simulink model "eVTOL_HIL"  (R2024b)
settings: Solver=FixedStepAuto  StartTime=0.0  StopTime=inf  FixedStep=SAMPLE_TIME  RelTol=1e-3
values from neighbouring files (symbols this model uses):
  aDl =     [initdata.mat]
  aDr =     [initdata.mat]
  aDyn =     [initdata.mat]
  aLat =     [initdata.mat]
  aLon =     [initdata.mat]
  D = Prop.D    [EOM_dt_MC.m]    (also in EOM_get_alf_dt_de_prop_evtol.m = CD * QS)
  General = init_layoutdata    [EOM_dt_MC.m]    (also in build_optimized_CA.m; initdata.mat = ; initdata_HIL_eVTOL.m)
  mass = Con(3)    [EOM_get_alf_dt_de_prop_evtol.m]    (also in initdata.mat = 2255.54; initdata_HIL_eVTOL.m = 7)
  Motor = init_motor_evtol    [EOM_dt_MC.m]    (also in initdata.mat = []; initdata_HIL_eVTOL.m)
  Prop = init_propeller_evtol_new    [EOM_dt_MC.m]    (also in initdata_HIL_eVTOL.m)
  SAMPLE_TIME = 0.01    [initdata_HIL_eVTOL.m]
undefined symbols (not defined in the file or in its folder): aDa, aDe, asbhl20env, Environment, InitData, magnitude
libraries: simulink_extras x16, vrlib x8, matrix_library x6, sharedutil x6, aerolibwindfilters x4, sharedtransform x4, aerolibfltsims x3, instrumentseriallib x3, uavmavlinklib x3, aerolibasang x3, aerolibobsolete x2, aerolibanimutils x1
(part 2 of 4)

== system eVTOL_HIL/eVTOL Dynamic Model/Environment/Wind Models ==
  Xe_x : Inport
  Ve : Inport  Port=2
  Altitude : Inport  Port=3
  DCM : Inport  Port=4
  Constant1 : Constant  Value=[0,0,0]
  Constant2 : Constant  Value=[0,0,0]
  Dot Product1 : DotProduct  OutDataTypeStr=Inherit: Inherit via internal rule
  Dot Product2 : DotProduct  OutDataTypeStr=Inherit: Inherit via internal rule
  Dryden Wind Turbulence Model (Continuous (+q -r)) : Subsystem  AncestorBlock=|  mask(Wind Turbulence Model){units=Metric (MKS), spec=MIL-F-8785C, model=Continuous Dryden (+q -r), W20=8, Wdeg=0, TurbProb=10^-4, L_high=533.4, Wingspan=7, ts=0.01, Seed=[23341 23342 23343 23344], T_on=on}
      | CustomLib_2019b/Dryden Wind Turbulence Model 
      | (Continuous (+q -r))
      mask prompts: units "aeroblks:aeroblkwind:blockWindTurbulenceModelParamUnits"; spec "aeroblks:aeroblkwind:blockWindTurbulenceModelParamSpecification"; model "aeroblks:aeroblkwind:blockWindTurbulenceModelParamModeltype"; W20 "Wind speed at 6 m defines the low-altitude intensity (m/s):"; Wdeg "Wind direction at 6 m (degrees clockwise from north):"; TurbProb "aeroblks:aeroblkwind:blockWindTurbulenceModelParamProbabilityofexceedanceofhighaltitudeintensity"; L_high "Scale length at medium/high altitudes (m):"; Wingspan "Wingspan (m):"; ts "Band limited noise sample time (sec):"; Seed "aeroblks:aeroblkwind:blockWindTurbulenceModelParamNoiseseedsugvgwgpg"; T_on "aeroblks:aeroblkwind:blockWindTurbulenceModelParamTurbulenceon"
      mask help: aeroblks:aeroblkwind:blockWindTurbulenceModelDesc
      mask init:
      | index = strfind(model,' ');
      | disp1 = model(1:index(1)-1);
      | disp2 = model(index(1)+1:index(end-1)-1);
      | disp3 = model(index(end-1)+1:end);
      | 
      | h_vec = [.5 1.75 3.75 7.5 15 25 35 45 55 65 75 80]*1000;% feet
      | sigma_vec(1,:) = [3.2 2.2 1.5 zeros(1,9)]; % ft/sec
      | sigma_vec(2,:) = [4.2 3.6 3.3 1.6 zeros(1,8)];
      | sigma_vec(3,:) = [6.6 6.9 7.4 6.7 4.6 2.7 0.4 zeros(1,5)];
      | sigma_vec(4,:) = [8.6 9.6 10.6 10.1 8.0 6.6 5.0 4.2 2.7 zeros(1,3)];
      | sigma_vec(5,:) = [11.8 13.0 16.0 15.1 11.6 9.7 8.1 8.2 7.9 4.9 3.2 2.1];
      | sigma_vec(6,:) = [15.6 17.6 23.0 23.6 22.1 20.0 16.0 15.1 12.1 7.9 6.2 5.1];
      | sigma_vec(7,:) = [18.7 21.5 28.4 30.2 30.7 31.0 25.2 23.1 17.5 10.7 8.4 7.2];
      | max_height_low = 1000;
      | if strcmp(spec,'MIL-F-8785C')
      |     min_height_high = 2000;
      | else
      | 	min_height_high = 1750;
      | end
      | [ports] = aeroicon('aeroblkwindturb2','icon');
      | 
      | dt=ts;
      settings: LibrarySourceBlock=|
      | CustomLib_2019b/Dryden Wind Turbulence Model
      | (Continuous (+q -r))
      mask Help: eval('asbhelp(''Dryden Wind Turbulence Model (Continuous)'')');
      mask TypeOptions units: aeroblks:aeroblkwind:blockWindTurbulenceModelParamComboMetricMKS | aeroblks:aeroblkwind:blockWindTurbulenceModelParamComboEnglishVelocityinfts | aeroblks:aeroblkwind:blockWindTurbulenceModelParamComboEnglishVelocityinkts
      mask TypeOptions spec: aeroblks:aeroblkwind:blockWindTurbulenceModelParamComboMILF8785C | aeroblks:aeroblkwind:blockWindTurbulenceModelParamComboMILHDBK1797 | aeroblks:aeroblkwind:blockWindTurbulenceModelParamComboMILHDBK1797B
      mask TypeOptions model: aeroblks:aeroblkwind:blockWindTurbulenceModelParamComboContinuousVonKarmanqr1 | aeroblks:aeroblkwind:blockWindTurbulenceModelParamComboContinuousVonKarmanqr2 | aeroblks:aeroblkwind:blockWindTurbulenceModelParamComboContinuousVonKarmanqr3 | aeroblks:aeroblkwind:blockWindTurbulenceModelParamComboContinuousDrydenqr1 | aeroblks:aeroblkwind:blockWindTurbulenceModelParamComboContinuousDrydenqr2 | aeroblks:aeroblkwind:blockWindTurbulenceModelParamComboContinuousDrydenqr3 | aeroblks:aeroblkwind:blockWindTurbulenceModelParamComboDiscreteDrydenqr1 | aeroblks:aeroblkwind:blockWindTurbulenceModelParamComboDiscreteDrydenqr2 | aeroblks:aeroblkwind:blockWindTurbulenceModelParamComboDiscreteDrydenqr3
      mask Callback model: aeroicon('aeroblkwindturb2');
      mask TypeOptions TurbProb: aeroblks:aeroblkwind:blockWindTurbulenceModelParamCombo2x101 | aeroblks:aeroblkwind:blockWindTurbulenceModelParamCombo101 | aeroblks:aeroblkwind:blockWindTurbulenceModelParamCombo102Light | aeroblks:aeroblkwind:blockWindTurbulenceModelParamCombo103Moderate | aeroblks:aeroblkwind:blockWindTurbulenceModelParamCombo104 | aeroblks:aeroblkwind:blockWindTurbulenceModelParamCombo105Severe | aeroblks:aeroblkwind:blockWindTurbulenceModelParamCombo106
      mask DialogControl units Prompt: Units:
      mask DialogControl spec Prompt: Specification:
      mask DialogControl model Prompt: Model type:
      mask DialogControl TurbProb Prompt: Probability of exceedance of high-altitude intensity:
      mask DialogControl Seed Prompt: Noise seeds [ug vg wg pg]:
      mask DialogControl T_on Prompt: Turbulence on
      mask Display:
      | port_label(ports(1).type,ports(1).port,ports(1).txt,'texmode','on');
      | port_label(ports(2).type,ports(2).port,ports(2).txt,'texmode','on');
      | port_label(ports(3).type,ports(3).port,ports(3).txt,'texmode','on');
      | port_label(ports(4).type,ports(4).port,ports(4).txt,'texmode','on');
      | port_label(ports(5).type,ports(5).port,ports(5).txt,'texmode','on');
  Gain4 : Gain  Gain=[1,1,1]
  Manual Switch1 : ManualSwitch  CurrentSetting=0
  Manual Switch2 : ManualSwitch  CurrentSetting=0
  Sqrt : Sqrt
  vt1 : Math  Operator=sqrt  SignedPower=on
  wind scp2 : Scope
  wind_mag scp : Scope
  windangular scp : Scope
  windspeed scp : Scope
  ug,vg,wg1 : Outport  VectorParamsAs1DForOutWhenUnconnected=off
  pg,qg,rg1 : Outport  Port=2  VectorParamsAs1DForOutWhenUnconnected=off
  wires:
  Manual Switch2/1 -> ug,vg,wg1/1  "WindVelocity"
  Dryden Wind Turbulence Model (Continuous (+q -r))/1(ug,vg,wg) -> Gain4/1, windspeed scp/1, Dot Product2/2, Dot Product2/1  "Vw"
  Dryden Wind Turbulence Model (Continuous (+q -r))/2(pg,qg,rg) -> Manual Switch1/1, windangular scp/1  "WindAngularRates"
  Constant1/1 -> Manual Switch1/2
  Altitude/1 -> [Altitude]
  vt1/1 -> [Airspeed]  "Airspeed"
  Constant2/1 -> Manual Switch2/2
  [Airspeed] -> Dryden Wind Turbulence Model (Continuous (+q -r))/2(Airspeed)  "Airspeed"
  DCM/1 -> [DCM]
  Ve/1 -> Dot Product1/2, Dot Product1/1
  Manual Switch1/1 -> pg,qg,rg1/1  "WindAngularRates"
  Gain4/1 -> Manual Switch2/1  "WindVelocity"
  [Altitude] -> Dryden Wind Turbulence Model (Continuous (+q -r))/1(Altitude)
  Dot Product2/1 -> Sqrt/1
  [DCM] -> Dryden Wind Turbulence Model (Continuous (+q -r))/3(DCM)
  Dot Product1/1 -> vt1/1
  Sqrt/1 -> wind_mag scp/1  "wind_mag"
  Xe_x/1 -> [x]
  [x] -> wind scp2/1

== system eVTOL_HIL/eVTOL Dynamic Model/airframe/Flight Conditions ==
  EnvData : Inport
  UAVData : Inport  Port=2
  Bus Selector : BusSelector  OutputSignals=Ve,Xe,Vb,pqr
  Bus Selector1 : BusSelector  OutputSignals=WindVelocity,WindAngularRate,T(K),a,Air_pressure,Air_density,g
  Constant : Constant  Value=0
  Demux1 : Demux  Outputs=2
  Derivative : Derivative
  Dynamic Pressure : aerolibasang/Dynamic Pressure
  Flat Earth to LLA : FlatEarth2LLA  R=6378137  LL0=[InitData.lat_deg, InitData.lon_deg]
  Gain : Gain  Gain=1/1.225
  "Incidence, Sideslip, & Airspeed" : aerolibasang/Incidence, Sideslip, & Airspeed
  MATLAB Function : MATLAB Function  TreatAsAtomicUnit=on
  Mach Number : aerolibasang/Mach Number
  Product : Product
  Sqrt : Sqrt
  Subsystem2 : Subsystem
  Sum : Sum  Inputs=|+-
  Sum1 : Sum  Inputs=|+-
  Vel in Inertial Axes : Subsystem
  lat_deg : Outport
  lon_deg : Outport  Port=2
  AMSL : Outport  Port=3
  gamma : Outport  Port=4
  chi : Outport  Port=5
  alphaDot : Outport  Port=6
  alpha : Outport  Port=7
  beta : Outport  Port=8
  TAS : Outport  Port=9
  pqr_air : Outport  Port=10
  Mach : Outport  Port=11
  DynamicPressure : Outport  Port=12
  EAS : Outport  Port=13
  T(K) : Outport  Port=14
  Air_pressure : Outport  Port=15
  g : Outport  Port=16
  Vb_air : Outport  Port=17
  Ve_Inertial : Outport  Port=18
  wires:
  Bus Selector/3 -> Sum/1  "<Vb>"
  Subsystem2/2(chi) -> chi/1  "chi"
  "Incidence, Sideslip, & Airspeed"/1 -> alpha/1, Derivative/1  "alpha"
  Subsystem2/1(gamma) -> gamma/1  "gamma"
  Demux1/1 -> lat_deg/1  "lat_deg"
  Bus Selector/2 -> Flat Earth to LLA/1  "<Xe>"
  Constant/1 -> Flat Earth to LLA/2
  Sum1/1 -> pqr_air/1  "pqr_air"
  Gain/1 -> Sqrt/1
  Flat Earth to LLA/2 -> AMSL/1  "AMSL"
  Product/1 -> EAS/1  "EAS"
  Bus Selector1/7 -> g/1  "<g>"
  Mach Number/1 -> Mach/1  "Mach"
  Bus Selector/4 -> Sum1/1  "<pqr>"
  UAVData/1 -> Bus Selector/1
  "Incidence, Sideslip, & Airspeed"/3 -> Product/1, TAS/1  "TAS"
  Bus Selector1/5 -> Air_pressure/1  "<Air_pressure>"
  Bus Selector1/6 -> Gain/1, Dynamic Pressure/2  "<Air_density>"
  Vel in Inertial Axes/1(Ve_Inertial) -> Ve_Inertial/1  "Ve_Inertial"
  Sum/1 -> "Incidence, Sideslip, & Airspeed"/1, Mach Number/1, Dynamic Pressure/1, MATLAB Function/1(u)  "Vb_air"
  Bus Selector1/3 -> T(K)/1  "<T(K)>"
  Derivative/1 -> alphaDot/1  "alphaDot"
  Bus Selector1/1 -> Sum/2  "<WindVelocity>"
  "Incidence, Sideslip, & Airspeed"/2 -> beta/1  "beta"
  Bus Selector/1 -> Vel in Inertial Axes/1(Ve), Subsystem2/1(Ve)  "<Ve>"
  Dynamic Pressure/1 -> DynamicPressure/1  "DynamicPressure"
  EnvData/1 -> Bus Selector1/1
  Bus Selector1/4 -> Mach Number/2  "<a>"
  Bus Selector1/2 -> Sum1/2  "<WindAngularRate>"
  Demux1/2 -> lon_deg/1  "lon_deg"
  Flat Earth to LLA/1 -> Demux1/1
  Sqrt/1 -> Product/2
  MATLAB Function/1(y) -> Vb_air/1

== system eVTOL_HIL/eVTOL Dynamic Model/airframe/force moment ==
  note: force and moment in body fixed axis coordination
  PlantData : Inport
  Act_surface : Inport  Port=2
  prop : Inport  Port=3
  EnvmData : Inport  Port=4
  Add : Sum  Inputs=++++
  Add1 : Sum  Inputs=++++
  Disturbance : Constant  Value=[0,10,0]
  Disturbance1 : Constant  Value=[0,0,0]
  F_Gear_in_b scp : Scope  Commented=on
  Gear&FM in body axis : Subsystem  Commented=on
  M_Gear scp : Scope  Commented=on
  Manual Switch : ManualSwitch  CurrentSetting=0
  Motor moment scp : Scope
  Scope{,1..4,6} (6 alike) : Scope
  Thrust&M in body axis : Subsystem
  aero F&M in body axis : Subsystem
  gravity in body axis : Subsystem
  Fb (X Y Z) : Outport  VectorParamsAs1DForOutWhenUnconnected=off
  M (L M N) : Outport  Port=2  VectorParamsAs1DForOutWhenUnconnected=off
  wires:
  Thrust&M in body axis/1(f_T) -> Add/1, Scope4/1
  gravity in body axis/1(Fb) -> Add/3, Scope3/1
  Thrust&M in body axis/2(m_T) -> Add1/1, Motor moment scp/1
  aero F&M in body axis/2(M (L M N)) -> Scope6/1, Add1/2
  Add1/1 -> Scope1/1, M (L M N)/1
  Add/1 -> Scope/1, Fb (X Y Z)/1
  PlantData/1 -> aero F&M in body axis/1(PlantData), Gear&FM in body axis/1(PlantData), gravity in body axis/1(PlantData)
  Act_surface/1 -> aero F&M in body axis/2(Act_surface)
  EnvmData/1 -> gravity in body axis/2(EnvmData)
  Gear&FM in body axis/1(F_Gear) -> Add/4, F_Gear_in_b scp/1
  Gear&FM in body axis/2(M_Gear) -> Add1/3, M_Gear scp/1
  aero F&M in body axis/1(Fb (X Y Z)) -> Add/2, Scope2/1
  Disturbance/1 -> Manual Switch/1
  Manual Switch/1 -> Add1/4
  Disturbance1/1 -> Manual Switch/2
  prop/1 -> Thrust&M in body axis/1(prop)

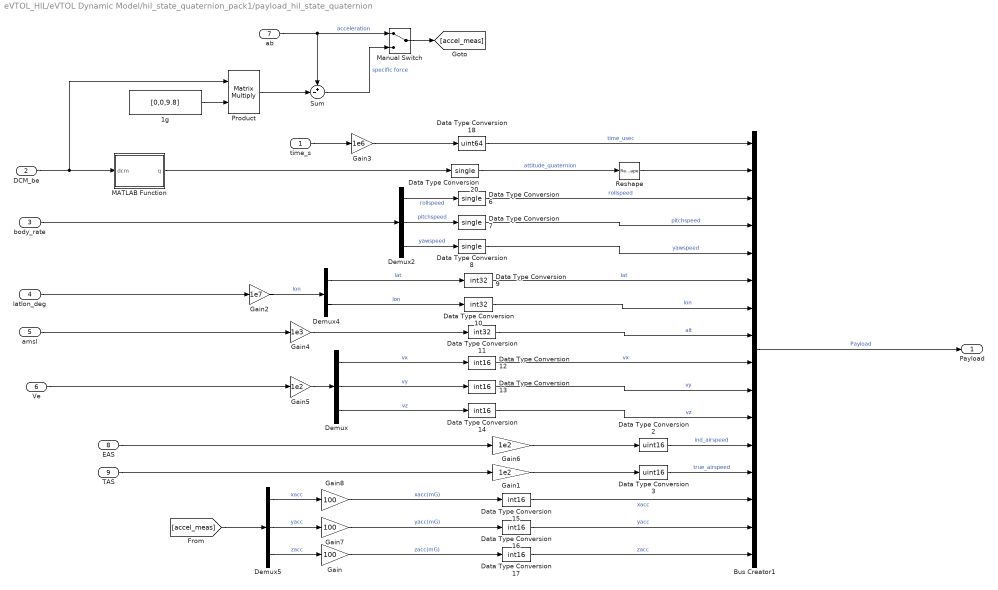
== system eVTOL_HIL/eVTOL Dynamic Model/hil_state_quaternion_pack1/payload_hil_state_quaternion ==
  time_s : Inport
  DCM_be : Inport  Port=2
  body_rate : Inport  Port=3
  latlon_deg : Inport  Port=4
  amsl : Inport  Port=5
  Ve : Inport  Port=6
  ab : Inport  Port=7
  EAS : Inport  Port=8
  TAS : Inport  Port=9
  1g : Constant  Value=[0,0,9.8]
  Bus Creator1 : BusCreator  Inputs=16
  Data Type Conversion10 : DataTypeConversion  OutDataTypeStr=int32  SaturateOnIntegerOverflow=off  RndMeth=Floor
  Data Type Conversion11 : DataTypeConversion  OutDataTypeStr=int32  SaturateOnIntegerOverflow=off  RndMeth=Floor
  Data Type Conversion{12..17} (6 alike) : DataTypeConversion  OutDataTypeStr=int16  SaturateOnIntegerOverflow=off  RndMeth=Floor
  Data Type Conversion18 : DataTypeConversion  OutDataTypeStr=uint64  SaturateOnIntegerOverflow=off  RndMeth=Floor
  Data Type Conversion2 : DataTypeConversion  OutDataTypeStr=uint16  SaturateOnIntegerOverflow=off  RndMeth=Floor
  Data Type Conversion{6..8,20} (4 alike) : DataTypeConversion  OutDataTypeStr=single  SaturateOnIntegerOverflow=off  RndMeth=Floor
  Data Type Conversion3 : DataTypeConversion  OutDataTypeStr=uint16  SaturateOnIntegerOverflow=off  RndMeth=Floor
  Data Type Conversion9 : DataTypeConversion  OutDataTypeStr=int32  SaturateOnIntegerOverflow=off  RndMeth=Floor
  Demux : Demux  Outputs=3
  Demux2 : Demux  Outputs=3
  Demux4 : Demux  Outputs=2
  Demux5 : Demux  Outputs=3
  Gain : Gain  Gain=100
  Gain1 : Gain  Gain=1e2
  Gain2 : Gain  Gain=1e7
  Gain3 : Gain  Gain=1e6
  Gain4 : Gain  Gain=1e3
  Gain5 : Gain  Gain=1e2
  Gain6 : Gain  Gain=1e2
  Gain7 : Gain  Gain=100
  Gain8 : Gain  Gain=100
  MATLAB Function : MATLAB Function  TreatAsAtomicUnit=on
  Manual Switch : ManualSwitch
  Product : Product  Multiplication=Matrix(*)
  Reshape : Reshape
  Sum : Sum  Inputs=+-|
  Payload : Outport
  wires:
  Manual Switch/1 -> [accel_meas]
  Sum/1 -> Manual Switch/2  "specific force"
  ab/1 -> Sum/1, Manual Switch/1  "acceleration"
  1g/1 -> Product/2
  Product/1 -> Sum/2
  Gain6/1 -> Data Type Conversion2/1
  EAS/1 -> Gain6/1
  Gain7/1 -> Data Type Conversion16/1  "yacc(mG)"
  Gain8/1 -> Data Type Conversion15/1  "xacc(mG)"
  Demux5/2 -> Gain7/1  "yacc"
  Demux5/1 -> Gain8/1  "xacc"
  Gain/1 -> Data Type Conversion17/1  "zacc(mG)"
  Demux5/3 -> Gain/1  "zacc"
  Data Type Conversion3/1 -> Bus Creator1/13  "true_airspeed"
  Data Type Conversion2/1 -> Bus Creator1/12  "ind_airspeed"
  Data Type Conversion20/1 -> Reshape/1  "attitude_quaternion"
  Gain1/1 -> Data Type Conversion3/1
  TAS/1 -> Gain1/1
  MATLAB Function/1(q) -> Data Type Conversion20/1
  Ve/1 -> Gain5/1
  Bus Creator1/1 -> Payload/1  "Payload"
  Data Type Conversion8/1 -> Bus Creator1/5  "yawspeed"
  DCM_be/1 -> MATLAB Function/1(dcm), Product/1
  latlon_deg/1 -> Gain2/1
  Demux/1 -> Data Type Conversion12/1  "vx"
  Data Type Conversion6/1 -> Bus Creator1/3  "rollspeed"
  [accel_meas] -> Demux5/1
  Data Type Conversion15/1 -> Bus Creator1/14  "xacc"
  Gain4/1 -> Data Type Conversion11/1
  body_rate/1 -> Demux2/1
  Data Type Conversion18/1 -> Bus Creator1/1  "time_usec"
  Gain3/1 -> Data Type Conversion18/1
  Demux4/1 -> Data Type Conversion9/1  "lat"
  Demux2/1 -> Data Type Conversion6/1  "rollspeed"
  time_s/1 -> Gain3/1
  Data Type Conversion12/1 -> Bus Creator1/9  "vx"
  Data Type Conversion17/1 -> Bus Creator1/16  "zacc"
  Data Type Conversion9/1 -> Bus Creator1/6  "lat"
  amsl/1 -> Gain4/1
  Data Type Conversion13/1 -> Bus Creator1/10  "vy"
  Gain2/1 -> Demux4/1  "lon"
  Data Type Conversion10/1 -> Bus Creator1/7  "lon"
  Demux2/3 -> Data Type Conversion8/1  "yawspeed"
  Demux/3 -> Data Type Conversion14/1  "vz"
  Demux/2 -> Data Type Conversion13/1  "vy"
  Gain5/1 -> Demux/1
  Demux4/2 -> Data Type Conversion10/1  "lon"
  Data Type Conversion16/1 -> Bus Creator1/15  "yacc"
  Data Type Conversion7/1 -> Bus Creator1/4  "pitchspeed"
  Demux2/2 -> Data Type Conversion7/1  "pitchspeed"
  Data Type Conversion14/1 -> Bus Creator1/11  "vz"
  Data Type Conversion11/1 -> Bus Creator1/8  "alt"
  Reshape/1 -> Bus Creator1/2

== system eVTOL_HIL/eVTOL Dynamic Model/Energy & Power/V_prop1/v_b to v_prop ==
  V_body : Inport
  i : Inport  Port=2
  Add : Sum  Inputs=+-
  Mux1 : Mux  Inputs=2
  Terminator : Terminator
  V_x : Fcn  Expr=u[1]*cos(u[4])
  V_y : Fcn  Expr=0
  V_z : Fcn  Expr=u[3]*sin(u[4])
  V : Outport  VectorParamsAs1DForOutWhenUnconnected=off
  wires:
  i/1 -> Mux1/2
  V_body/1 -> Mux1/1
  Mux1/1 -> V_z/1, V_y/1, V_x/1
  Add/1 -> V/1
  V_x/1 -> Add/1
  V_z/1 -> Add/2
  V_y/1 -> Terminator/1

== system eVTOL_HIL/eVTOL Dynamic Model/Energy & Power/V_prop2/v_b to v_prop ==
  V_body : Inport
  i : Inport  Port=2
  Add : Sum  Inputs=+-
  Mux1 : Mux  Inputs=2
  Terminator : Terminator
  V_x : Fcn  Expr=u[1]*cos(u[4])
  V_y : Fcn  Expr=0
  V_z : Fcn  Expr=u[3]*sin(u[4])
  V : Outport  VectorParamsAs1DForOutWhenUnconnected=off
  wires:
  i/1 -> Mux1/2
  V_body/1 -> Mux1/1
  Mux1/1 -> V_z/1, V_y/1, V_x/1
  V_z/1 -> Add/2
  V_x/1 -> Add/1
  Add/1 -> V/1
  V_y/1 -> Terminator/1

== system eVTOL_HIL/eVTOL Dynamic Model/Energy & Power/V_prop3/v_b to v_prop ==
  V_body : Inport
  i : Inport  Port=2
  Add : Sum  Inputs=+-
  Mux1 : Mux  Inputs=2
  Terminator : Terminator
  V_x : Fcn  Expr=u[1]*cos(u[4])
  V_y : Fcn  Expr=0
  V_z : Fcn  Expr=u[3]*sin(u[4])
  V : Outport  VectorParamsAs1DForOutWhenUnconnected=off
  wires:
  i/1 -> Mux1/2
  V_body/1 -> Mux1/1
  Mux1/1 -> V_z/1, V_y/1, V_x/1
  V_z/1 -> Add/2
  V_x/1 -> Add/1
  Add/1 -> V/1
  V_y/1 -> Terminator/1

== system eVTOL_HIL/eVTOL Dynamic Model/Energy & Power/V_prop4/v_b to v_prop ==
  V_body : Inport
  i : Inport  Port=2
  Add : Sum  Inputs=+-
  Mux1 : Mux  Inputs=2
  Terminator : Terminator
  V_x : Fcn  Expr=u[1]*cos(u[4])
  V_y : Fcn  Expr=0
  V_z : Fcn  Expr=u[3]*sin(u[4])
  V : Outport  VectorParamsAs1DForOutWhenUnconnected=off
  wires:
  i/1 -> Mux1/2
  V_body/1 -> Mux1/1
  Mux1/1 -> V_z/1, V_y/1, V_x/1
  V_x/1 -> Add/1
  Add/1 -> V/1
  V_z/1 -> Add/2
  V_y/1 -> Terminator/1

== system eVTOL_HIL/eVTOL Dynamic Model/Energy & Power/V_prop5/v_b to v_prop ==
  V_body : Inport
  i : Inport  Port=2
  Add : Sum  Inputs=+-
  Mux1 : Mux  Inputs=2
  Terminator : Terminator
  V_x : Fcn  Expr=u[1]*cos(u[4])
  V_y : Fcn  Expr=0
  V_z : Fcn  Expr=u[3]*sin(u[4])
  V : Outport  VectorParamsAs1DForOutWhenUnconnected=off
  wires:
  i/1 -> Mux1/2
  V_body/1 -> Mux1/1
  Mux1/1 -> V_z/1, V_y/1, V_x/1
  V_z/1 -> Add/2
  V_x/1 -> Add/1
  Add/1 -> V/1
  V_y/1 -> Terminator/1

== system eVTOL_HIL/eVTOL Dynamic Model/Energy & Power/V_prop6/v_b to v_prop ==
  V_body : Inport
  i : Inport  Port=2
  Add : Sum  Inputs=+-
  Mux1 : Mux  Inputs=2
  Terminator : Terminator
  V_x : Fcn  Expr=u[1]*cos(u[4])
  V_y : Fcn  Expr=0
  V_z : Fcn  Expr=u[3]*sin(u[4])
  V : Outport  VectorParamsAs1DForOutWhenUnconnected=off
  wires:
  i/1 -> Mux1/2
  V_body/1 -> Mux1/1
  Mux1/1 -> V_z/1, V_y/1, V_x/1
  V_z/1 -> Add/2
  V_x/1 -> Add/1
  Add/1 -> V/1
  V_y/1 -> Terminator/1

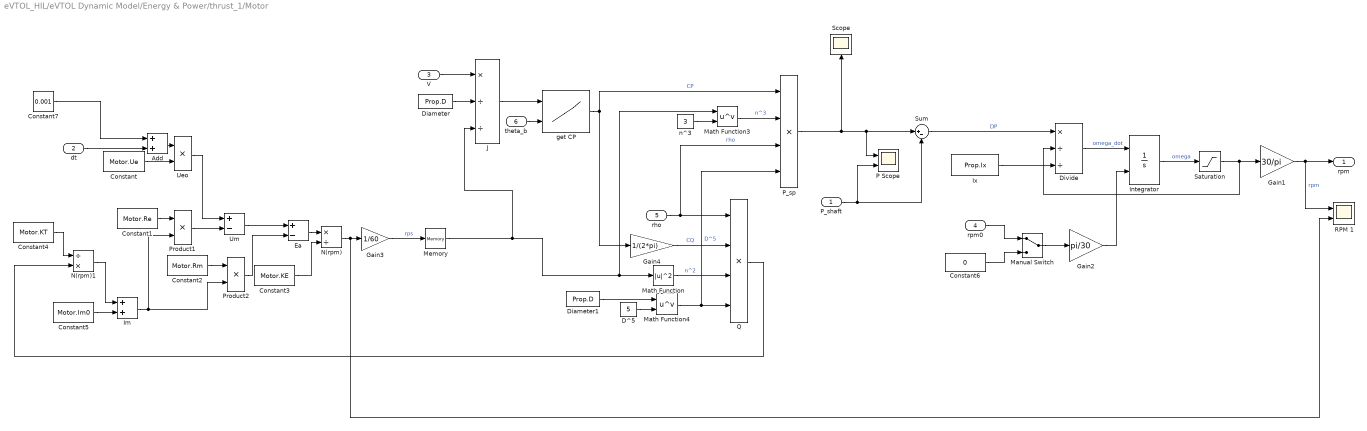
== system eVTOL_HIL/eVTOL Dynamic Model/Energy & Power/thrust_1/Motor ==
  P_shaft : Inport
  dt : Inport  Port=2
  V : Inport  Port=3
  rpm0 : Inport  Port=4
  rho : Inport  Port=5
  theta_b : Inport  Port=6
  Add : Sum
  Constant : Constant  Value=Motor.Ue
  Constant1 : Constant  Value=Motor.Re
  Constant2 : Constant  Value=Motor.Rm
  Constant3 : Constant  Value=Motor.KE
  Constant4 : Constant  Value=Motor.KT  VectorParams1D=off
  Constant5 : Constant  Value=Motor.Im0
  Constant6 : Constant  Value=0
  Constant7 : Constant  Value=0.001
  D^5 : Constant  Value=5
  Diameter : Constant  Value=Prop.D
  Diameter1 : Constant  Value=Prop.D
  Divide : Product  Inputs=*//
  Ea : Sum  Inputs=+-
  Gain1 : Gain  Gain=30/pi
  Gain2 : Gain  Gain=pi/30
  Gain3 : Gain  Gain=1/60
  Gain4 : Gain  Gain=1/(2*pi)
  Im : Sum
  Integrator : Integrator  InitialConditionSource=external  InitialCondition=600
  Ix : Constant  Value=Prop.Ix
  J : Product  Inputs=*//
  Manual Switch : ManualSwitch
  Math Function : Math  Operator=magnitude^2  SignedPower=on
  Math Function3 : Math  Operator=pow  SignedPower=on
  Math Function4 : Math  Operator=pow  SignedPower=on
  Memory : Memory  InitialCondition=0.1
  N(rpm) : Product  Inputs=*/
  N(rpm)1 : Product  Inputs=/*
  P Scope : Scope  NumInputPorts=2
  P_sp : Product  Inputs=4
  Product1 : Product
  Product2 : Product
  Q : Product  Inputs=4
  RPM 1 : Scope  NumInputPorts=2
  Saturation : Saturate  UpperLimit=104.72  LowerLimit=0.1
  Scope : Scope
  Sum : Sum  Inputs=|+-
  Ueo : Product
  Um : Sum  Inputs=+-
  get CP : Lookup_n-D  BreakpointsForDimension1=Prop.J  BreakpointsForDimension2=Prop.theta_b  IndexSearchMethod=Linear search  BeginIndexSearchUsingPreviousIndexResult=on  Table=Prop.CP  RndMeth=Simplest
      settings: InputPortMap=u0,u1
  "n^3 " : Constant  Value=3
  rpm : Outport  VectorParamsAs1DForOutWhenUnconnected=off
  wires:
  Saturation/1 -> Gain1/1, Divide/2
  Gain2/1 -> Integrator/2
  rpm0/1 -> Manual Switch/1
  Gain1/1 -> rpm/1, RPM 1/1  "rpm"
  Sum/1 -> Divide/1  "DP"
  Divide/1 -> Integrator/1  "omega_dot"
  Integrator/1 -> Saturation/1  "omega"
  P_sp/1 -> Scope/1, P Scope/1, Sum/1
  P_shaft/1 -> P Scope/2, Sum/2
  Ix/1 -> Divide/3
  Constant/1 -> Ueo/2
  Ueo/1 -> Um/1
  Product1/1 -> Um/2
  Constant1/1 -> Product1/1
  Um/1 -> Ea/1
  Product2/1 -> Ea/2
  Constant2/1 -> Product2/1
  Ea/1 -> N(rpm)/1
  Constant3/1 -> N(rpm)/2
  Diameter/1 -> J/2
  V/1 -> J/1
  N(rpm)/1 -> Gain3/1, RPM 1/2
  J/1 -> get CP/1
  theta_b/1 -> get CP/2
  Gain4/1 -> Q/2  "CQ"
  D^5/1 -> Math Function4/2
  Diameter1/1 -> Math Function4/1
  Math Function/1 -> Q/3  "n^2"
  Q/1 -> N(rpm)1/2
  Constant4/1 -> N(rpm)1/1
  N(rpm)1/1 -> Im/1
  Constant5/1 -> Im/2
  Im/1 -> Product2/2, Product1/2
  rho/1 -> Q/1, P_sp/3  "rho"
  Math Function3/1 -> P_sp/2  "n^3"
  "n^3 "/1 -> Math Function3/2
  Math Function4/1 -> Q/4, P_sp/4  "D^5"
  get CP/1 -> Gain4/1, P_sp/1  "CP"
  Manual Switch/1 -> Gain2/1
  Constant6/1 -> Manual Switch/2
  Constant7/1 -> Add/1
  Add/1 -> Ueo/1
  dt/1 -> Add/2
  Gain3/1 -> Memory/1  "rps"
  Memory/1 -> J/3, Math Function3/1, Math Function/1

== system eVTOL_HIL/eVTOL Dynamic Model/Energy & Power/thrust_1/Propeller  ==
  rpm : Inport
  V : Inport  Port=2
  rho : Inport  Port=3
  theta_b : Inport  Port=4
  D^5 : Constant  Value=5
  Diameter : Constant  Value=Prop.D
  Display1 : Display
  Display7 : Display
  Divide : Product  Inputs=4
  Divide2 : Product  Inputs=4
  Divide3 : Product  Inputs=**/
  Gain : Gain  Gain=1/60
  Math Function : Math  Operator=magnitude^2  SignedPower=on
  Math Function1 : Math  Operator=magnitude^2  SignedPower=on
  Math Function2 : Math  Operator=magnitude^2  SignedPower=on
  Math Function3 : Math  Operator=pow  SignedPower=on
  Math Function4 : Math  Operator=pow  SignedPower=on
  Scope{,1..4} (5 alike) : Scope
  Subsystem : Subsystem
  get CP : Lookup_n-D  BreakpointsForDimension1=Prop.J  BreakpointsForDimension2=Prop.theta_b  IndexSearchMethod=Linear search  BeginIndexSearchUsingPreviousIndexResult=on  Table=Prop.CP  RndMeth=Simplest
      settings: InputPortMap=u0,u1
  get CT : Lookup_n-D  BreakpointsForDimension1=Prop.J  BreakpointsForDimension2=Prop.theta_b  IndexSearchMethod=Linear search  BeginIndexSearchUsingPreviousIndexResult=on  Table=Prop.CT  RndMeth=Simplest
      settings: InputPortMap=u0,u1
  "n^3 " : Constant  Value=3
  P_plr (w) : Outport  VectorParamsAs1DForOutWhenUnconnected=off
  T (N) : Outport  Port=2  VectorParamsAs1DForOutWhenUnconnected=off
  eta_p : Outport  Port=3  VectorParamsAs1DForOutWhenUnconnected=off
  wires:
  Divide2/1 -> Scope/1, P_plr (w)/1
  Divide3/1 -> eta_p/1  "eta_p"
  D^5/1 -> Math Function4/2
  Math Function4/1 -> Divide2/4
  "n^3 "/1 -> Math Function3/2
  Math Function3/1 -> Divide2/3
  get CP/1 -> Display1/1, Divide3/3, Divide2/1, Scope3/1
  rpm/1 -> Gain/1, Subsystem/2(rpm)
  Subsystem/1(J) -> Scope2/1, get CT/1, Divide3/1, get CP/1
  Divide/1 -> Scope1/1, T (N)/1
  Math Function2/1 -> Divide/4  "D^4"
  Math Function1/1 -> Math Function2/1
  Diameter/1 -> Math Function1/1, Math Function4/1
  Math Function/1 -> Divide/3  "n^2"
  Gain/1 -> Math Function3/1, Math Function/1
  rho/1 -> Divide/2, Divide2/2
  get CT/1 -> Display7/1, Divide3/2, Divide/1, Scope4/1
  V/1 -> Subsystem/1(V)
  theta_b/1 -> get CP/2, get CT/2

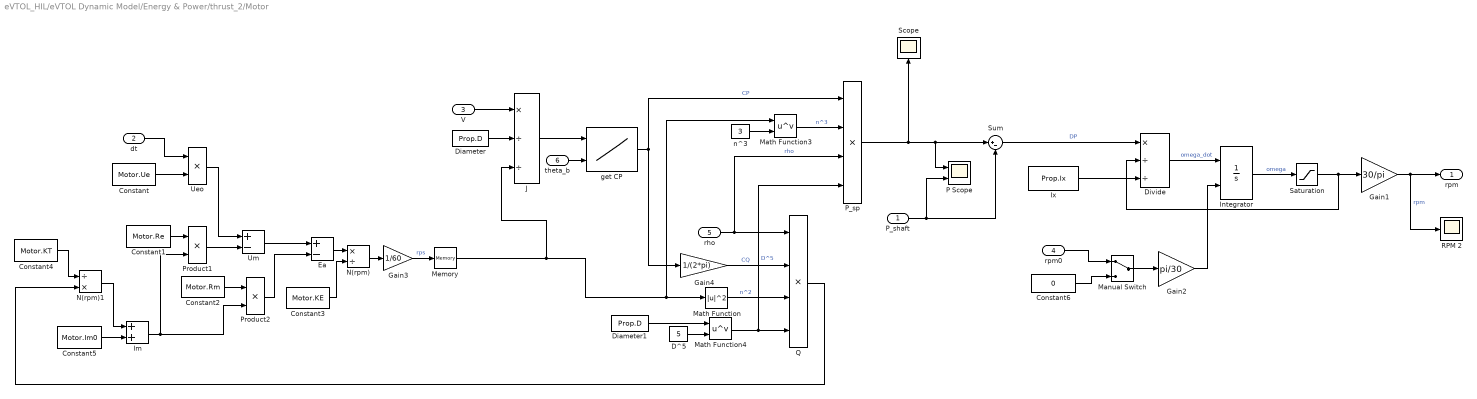
== system eVTOL_HIL/eVTOL Dynamic Model/Energy & Power/thrust_2/Motor ==
  P_shaft : Inport
  dt : Inport  Port=2
  V : Inport  Port=3
  rpm0 : Inport  Port=4
  rho : Inport  Port=5
  theta_b : Inport  Port=6
  Constant : Constant  Value=Motor.Ue
  Constant1 : Constant  Value=Motor.Re
  Constant2 : Constant  Value=Motor.Rm
  Constant3 : Constant  Value=Motor.KE
  Constant4 : Constant  Value=Motor.KT  VectorParams1D=off
  Constant5 : Constant  Value=Motor.Im0
  Constant6 : Constant  Value=0
  D^5 : Constant  Value=5
  Diameter : Constant  Value=Prop.D
  Diameter1 : Constant  Value=Prop.D
  Divide : Product  Inputs=*//
  Ea : Sum  Inputs=+-
  Gain1 : Gain  Gain=30/pi
  Gain2 : Gain  Gain=pi/30
  Gain3 : Gain  Gain=1/60
  Gain4 : Gain  Gain=1/(2*pi)
  Im : Sum
  Integrator : Integrator  InitialConditionSource=external  InitialCondition=600
  Ix : Constant  Value=Prop.Ix
  J : Product  Inputs=*//
  Manual Switch : ManualSwitch
  Math Function : Math  Operator=magnitude^2  SignedPower=on
  Math Function3 : Math  Operator=pow  SignedPower=on
  Math Function4 : Math  Operator=pow  SignedPower=on
  Memory : Memory  InitialCondition=0.1
  N(rpm) : Product  Inputs=*/
  N(rpm)1 : Product  Inputs=/*
  P Scope : Scope  NumInputPorts=2
  P_sp : Product  Inputs=4
  Product1 : Product
  Product2 : Product
  Q : Product  Inputs=4
  RPM 2 : Scope
  Saturation : Saturate  UpperLimit=104.72  LowerLimit=0.1
  Scope : Scope
  Sum : Sum  Inputs=|+-
  Ueo : Product
  Um : Sum  Inputs=+-
  get CP : Lookup_n-D  BreakpointsForDimension1=Prop.J  BreakpointsForDimension2=Prop.theta_b  IndexSearchMethod=Linear search  BeginIndexSearchUsingPreviousIndexResult=on  Table=Prop.CP  RndMeth=Simplest
      settings: InputPortMap=u0,u1
  "n^3 " : Constant  Value=3
  rpm : Outport  VectorParamsAs1DForOutWhenUnconnected=off
  wires:
  Saturation/1 -> Gain1/1, Divide/2
  Gain2/1 -> Integrator/2
  rpm0/1 -> Manual Switch/1
  Gain1/1 -> rpm/1, RPM 2/1  "rpm"
  Sum/1 -> Divide/1  "DP"
  Divide/1 -> Integrator/1  "omega_dot"
  dt/1 -> Ueo/1
  Integrator/1 -> Saturation/1  "omega"
  P_sp/1 -> Scope/1, P Scope/1, Sum/1
  P_shaft/1 -> P Scope/2, Sum/2
  Ix/1 -> Divide/3
  Constant/1 -> Ueo/2
  Ueo/1 -> Um/1
  Product1/1 -> Um/2
  Constant1/1 -> Product1/1
  Um/1 -> Ea/1
  Product2/1 -> Ea/2
  Constant2/1 -> Product2/1
  Ea/1 -> N(rpm)/1
  Constant3/1 -> N(rpm)/2
  Diameter/1 -> J/2
  V/1 -> J/1
  N(rpm)/1 -> Gain3/1
  J/1 -> get CP/1
  theta_b/1 -> get CP/2
  Gain4/1 -> Q/2  "CQ"
  D^5/1 -> Math Function4/2
  Diameter1/1 -> Math Function4/1
  Math Function/1 -> Q/3  "n^2"
  Q/1 -> N(rpm)1/2
  Constant4/1 -> N(rpm)1/1
  N(rpm)1/1 -> Im/1
  Constant5/1 -> Im/2
  Im/1 -> Product2/2, Product1/2
  rho/1 -> Q/1, P_sp/3  "rho"
  Math Function3/1 -> P_sp/2  "n^3"
  "n^3 "/1 -> Math Function3/2
  Math Function4/1 -> Q/4, P_sp/4  "D^5"
  get CP/1 -> Gain4/1, P_sp/1  "CP"
  Constant6/1 -> Manual Switch/2
  Manual Switch/1 -> Gain2/1
  Gain3/1 -> Memory/1  "rps"
  Memory/1 -> J/3, Math Function3/1, Math Function/1

== system eVTOL_HIL/eVTOL Dynamic Model/Energy & Power/thrust_2/Propeller  ==
  rpm : Inport
  V : Inport  Port=2
  rho : Inport  Port=3
  theta_b : Inport  Port=4
  D^5 : Constant  Value=5
  Diameter : Constant  Value=Prop.D
  Divide : Product  Inputs=4
  Divide2 : Product  Inputs=4
  Divide3 : Product  Inputs=**/
  Gain : Gain  Gain=1/60
  Math Function : Math  Operator=magnitude^2  SignedPower=on
  Math Function1 : Math  Operator=magnitude^2  SignedPower=on
  Math Function2 : Math  Operator=magnitude^2  SignedPower=on
  Math Function3 : Math  Operator=pow  SignedPower=on
  Math Function4 : Math  Operator=pow  SignedPower=on
  Scope{,1..4} (5 alike) : Scope
  Subsystem : Subsystem
  get CP : Lookup_n-D  BreakpointsForDimension1=Prop.J  BreakpointsForDimension2=Prop.theta_b  IndexSearchMethod=Linear search  BeginIndexSearchUsingPreviousIndexResult=on  Table=Prop.CP  RndMeth=Simplest
      settings: InputPortMap=u0,u1
  get CT : Lookup_n-D  BreakpointsForDimension1=Prop.J  BreakpointsForDimension2=Prop.theta_b  IndexSearchMethod=Linear search  BeginIndexSearchUsingPreviousIndexResult=on  Table=Prop.CT  RndMeth=Simplest
      settings: InputPortMap=u0,u1
  "n^3 " : Constant  Value=3
  P_plr (w) : Outport  VectorParamsAs1DForOutWhenUnconnected=off
  T (N) : Outport  Port=2  VectorParamsAs1DForOutWhenUnconnected=off
  eta_p : Outport  Port=3  VectorParamsAs1DForOutWhenUnconnected=off
  wires:
  Divide2/1 -> P_plr (w)/1, Scope/1
  Divide3/1 -> eta_p/1  "eta_p"
  D^5/1 -> Math Function4/2
  Math Function4/1 -> Divide2/4
  "n^3 "/1 -> Math Function3/2
  Math Function3/1 -> Divide2/3
  get CP/1 -> Divide3/3, Divide2/1, Scope3/1
  rpm/1 -> Gain/1, Subsystem/2(rpm)
  Subsystem/1(J) -> Scope2/1, get CT/1, Divide3/1, get CP/1
  Divide/1 -> Scope1/1, T (N)/1
  Math Function2/1 -> Divide/4  "D^4"
  Math Function1/1 -> Math Function2/1
  Diameter/1 -> Math Function1/1, Math Function4/1
  Math Function/1 -> Divide/3  "n^2"
  Gain/1 -> Math Function3/1, Math Function/1
  rho/1 -> Divide/2, Divide2/2
  get CT/1 -> Divide3/2, Divide/1, Scope4/1
  V/1 -> Subsystem/1(V)
  theta_b/1 -> get CP/2, get CT/2

== system eVTOL_HIL/eVTOL Dynamic Model/Energy & Power/thrust_3/Motor ==
  P_shaft : Inport
  dt : Inport  Port=2
  V : Inport  Port=3
  rpm0 : Inport  Port=4
  rho : Inport  Port=5
  theta_b : Inport  Port=6
  Constant : Constant  Value=Motor.Ue
  Constant1 : Constant  Value=Motor.Re
  Constant2 : Constant  Value=Motor.Rm
  Constant3 : Constant  Value=Motor.KE
  Constant4 : Constant  Value=Motor.KT  VectorParams1D=off
  Constant5 : Constant  Value=Motor.Im0
  Constant6 : Constant  Value=0
  D^5 : Constant  Value=5
  Diameter : Constant  Value=Prop.D
  Diameter1 : Constant  Value=Prop.D
  Divide : Product  Inputs=*//
  Ea : Sum  Inputs=+-
  Gain1 : Gain  Gain=30/pi
  Gain2 : Gain  Gain=pi/30
  Gain3 : Gain  Gain=1/60
  Gain4 : Gain  Gain=1/(2*pi)
  Im : Sum
  Integrator : Integrator  InitialConditionSource=external  InitialCondition=600
  Ix : Constant  Value=Prop.Ix
  J : Product  Inputs=*//
  Manual Switch : ManualSwitch
  Math Function : Math  Operator=magnitude^2  SignedPower=on
  Math Function3 : Math  Operator=pow  SignedPower=on
  Math Function4 : Math  Operator=pow  SignedPower=on
  Memory : Memory  InitialCondition=0.1
  N(rpm) : Product  Inputs=*/
  N(rpm)1 : Product  Inputs=/*
  P Scope : Scope  NumInputPorts=2
  P_sp : Product  Inputs=4
  Product1 : Product
  Product2 : Product
  Q : Product  Inputs=4
  RPM 3 : Scope
  Saturation : Saturate  UpperLimit=104.72  LowerLimit=0.1
  Scope : Scope
  Sum : Sum  Inputs=|+-
  Ueo : Product
  Um : Sum  Inputs=+-
  get CP : Lookup_n-D  BreakpointsForDimension1=Prop.J  BreakpointsForDimension2=Prop.theta_b  IndexSearchMethod=Linear search  BeginIndexSearchUsingPreviousIndexResult=on  Table=Prop.CP  RndMeth=Simplest
      settings: InputPortMap=u0,u1
  "n^3 " : Constant  Value=3
  rpm : Outport  VectorParamsAs1DForOutWhenUnconnected=off
  wires:
  Saturation/1 -> Gain1/1, Divide/2
  Gain2/1 -> Integrator/2
  rpm0/1 -> Manual Switch/1
  Gain1/1 -> rpm/1, RPM 3/1  "rpm"
  Sum/1 -> Divide/1  "DP"
  Divide/1 -> Integrator/1  "omega_dot"
  dt/1 -> Ueo/1
  Integrator/1 -> Saturation/1  "omega"
  P_sp/1 -> Scope/1, P Scope/1, Sum/1
  P_shaft/1 -> P Scope/2, Sum/2
  Ix/1 -> Divide/3
  Constant/1 -> Ueo/2
  Ueo/1 -> Um/1
  Product1/1 -> Um/2
  Constant1/1 -> Product1/1
  Um/1 -> Ea/1
  Product2/1 -> Ea/2
  Constant2/1 -> Product2/1
  Ea/1 -> N(rpm)/1
  Constant3/1 -> N(rpm)/2
  Diameter/1 -> J/2
  V/1 -> J/1
  N(rpm)/1 -> Gain3/1
  J/1 -> get CP/1
  theta_b/1 -> get CP/2
  Gain4/1 -> Q/2  "CQ"
  D^5/1 -> Math Function4/2
  Diameter1/1 -> Math Function4/1
  Math Function/1 -> Q/3  "n^2"
  Q/1 -> N(rpm)1/2
  Constant4/1 -> N(rpm)1/1
  N(rpm)1/1 -> Im/1
  Constant5/1 -> Im/2
  Im/1 -> Product1/2, Product2/2
  rho/1 -> Q/1, P_sp/3  "rho"
  Math Function3/1 -> P_sp/2  "n^3"
  "n^3 "/1 -> Math Function3/2
  Math Function4/1 -> Q/4, P_sp/4  "D^5"
  get CP/1 -> Gain4/1, P_sp/1  "CP"
  Constant6/1 -> Manual Switch/2
  Manual Switch/1 -> Gain2/1
  Gain3/1 -> Memory/1  "rps"
  Memory/1 -> J/3, Math Function3/1, Math Function/1

== system eVTOL_HIL/eVTOL Dynamic Model/Energy & Power/thrust_3/Propeller  ==
  rpm : Inport
  V : Inport  Port=2
  rho : Inport  Port=3
  theta_b : Inport  Port=4
  D^5 : Constant  Value=5
  Diameter : Constant  Value=Prop.D
  Divide : Product  Inputs=4
  Divide2 : Product  Inputs=4
  Divide3 : Product  Inputs=**/
  Gain : Gain  Gain=1/60
  Math Function : Math  Operator=magnitude^2  SignedPower=on
  Math Function1 : Math  Operator=magnitude^2  SignedPower=on
  Math Function2 : Math  Operator=magnitude^2  SignedPower=on
  Math Function3 : Math  Operator=pow  SignedPower=on
  Math Function4 : Math  Operator=pow  SignedPower=on
  Scope{,1..4} (5 alike) : Scope
  Subsystem : Subsystem
  get CP : Lookup_n-D  BreakpointsForDimension1=Prop.J  BreakpointsForDimension2=Prop.theta_b  IndexSearchMethod=Linear search  BeginIndexSearchUsingPreviousIndexResult=on  Table=Prop.CP  RndMeth=Simplest
      settings: InputPortMap=u0,u1
  get CT : Lookup_n-D  BreakpointsForDimension1=Prop.J  BreakpointsForDimension2=Prop.theta_b  IndexSearchMethod=Linear search  BeginIndexSearchUsingPreviousIndexResult=on  Table=Prop.CT  RndMeth=Simplest
      settings: InputPortMap=u0,u1
  "n^3 " : Constant  Value=3
  P_plr (w) : Outport  VectorParamsAs1DForOutWhenUnconnected=off
  T (N) : Outport  Port=2  VectorParamsAs1DForOutWhenUnconnected=off
  eta_p : Outport  Port=3  VectorParamsAs1DForOutWhenUnconnected=off
  wires:
  Divide2/1 -> P_plr (w)/1, Scope/1
  Divide3/1 -> eta_p/1  "eta_p"
  D^5/1 -> Math Function4/2
  Math Function4/1 -> Divide2/4
  "n^3 "/1 -> Math Function3/2
  Math Function3/1 -> Divide2/3
  get CP/1 -> Divide3/3, Divide2/1, Scope3/1
  rpm/1 -> Gain/1, Subsystem/2(rpm)
  Subsystem/1(J) -> Scope2/1, get CT/1, Divide3/1, get CP/1
  Divide/1 -> Scope1/1, T (N)/1
  Math Function2/1 -> Divide/4  "D^4"
  Math Function1/1 -> Math Function2/1
  Diameter/1 -> Math Function1/1, Math Function4/1
  Math Function/1 -> Divide/3  "n^2"
  Gain/1 -> Math Function3/1, Math Function/1
  rho/1 -> Divide/2, Divide2/2
  get CT/1 -> Divide3/2, Divide/1, Scope4/1
  V/1 -> Subsystem/1(V)
  theta_b/1 -> get CP/2, get CT/2

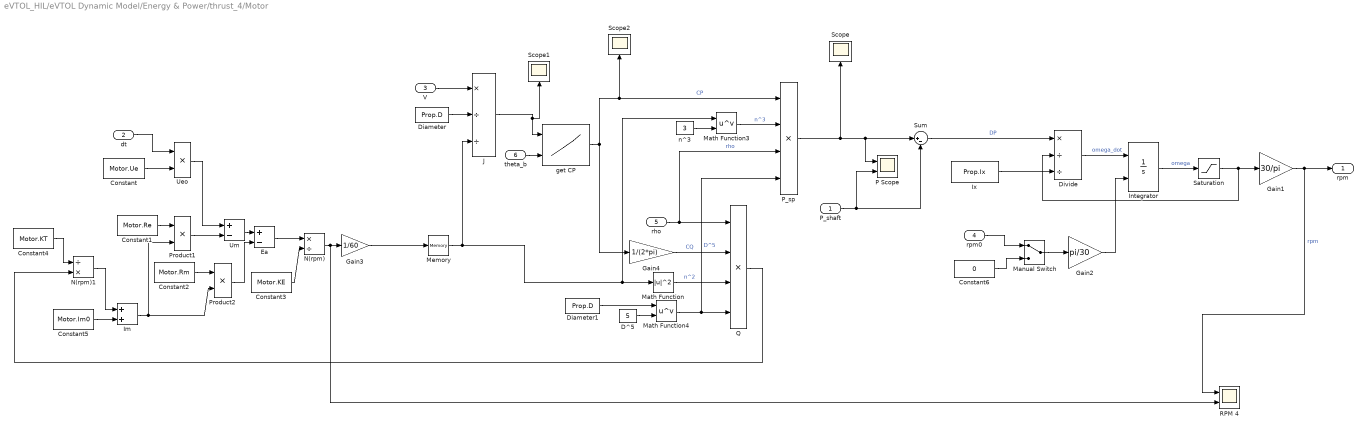
== system eVTOL_HIL/eVTOL Dynamic Model/Energy & Power/thrust_4/Motor ==
  P_shaft : Inport
  dt : Inport  Port=2
  V : Inport  Port=3
  rpm0 : Inport  Port=4
  rho : Inport  Port=5
  theta_b : Inport  Port=6
  Constant : Constant  Value=Motor.Ue
  Constant1 : Constant  Value=Motor.Re
  Constant2 : Constant  Value=Motor.Rm
  Constant3 : Constant  Value=Motor.KE
  Constant4 : Constant  Value=Motor.KT  VectorParams1D=off
  Constant5 : Constant  Value=Motor.Im0
  Constant6 : Constant  Value=0
  D^5 : Constant  Value=5
  Diameter : Constant  Value=Prop.D
  Diameter1 : Constant  Value=Prop.D
  Divide : Product  Inputs=*//
  Ea : Sum  Inputs=+-
  Gain1 : Gain  Gain=30/pi
  Gain2 : Gain  Gain=pi/30
  Gain3 : Gain  Gain=1/60
  Gain4 : Gain  Gain=1/(2*pi)
  Im : Sum
  Integrator : Integrator  InitialConditionSource=external  InitialCondition=600
  Ix : Constant  Value=Prop.Ix
  J : Product  Inputs=*//
  Manual Switch : ManualSwitch
  Math Function : Math  Operator=magnitude^2  SignedPower=on
  Math Function3 : Math  Operator=pow  SignedPower=on
  Math Function4 : Math  Operator=pow  SignedPower=on
  Memory : Memory  InitialCondition=0.1
  N(rpm) : Product  Inputs=*/
  N(rpm)1 : Product  Inputs=/*
  P Scope : Scope  NumInputPorts=2
  P_sp : Product  Inputs=4
  Product1 : Product
  Product2 : Product
  Q : Product  Inputs=4
  RPM 4 : Scope  NumInputPorts=2
  Saturation : Saturate  UpperLimit=104.72  LowerLimit=0.1
  Scope : Scope
  Scope1 : Scope
  Scope2 : Scope
  Sum : Sum  Inputs=|+-
  Ueo : Product
  Um : Sum  Inputs=+-
  get CP : Lookup_n-D  BreakpointsForDimension1=Prop.J  BreakpointsForDimension2=Prop.theta_b  IndexSearchMethod=Linear search  BeginIndexSearchUsingPreviousIndexResult=on  Table=Prop.CP  RndMeth=Simplest
      settings: InputPortMap=u0,u1
  "n^3 " : Constant  Value=3
  rpm : Outport  VectorParamsAs1DForOutWhenUnconnected=off
  wires:
  Saturation/1 -> Gain1/1, Divide/2
  Gain2/1 -> Integrator/2
  rpm0/1 -> Manual Switch/1
  Gain1/1 -> rpm/1, RPM 4/1  "rpm"
  Sum/1 -> Divide/1  "DP"
  Divide/1 -> Integrator/1  "omega_dot"
  dt/1 -> Ueo/1
  Integrator/1 -> Saturation/1  "omega"
  P_sp/1 -> Scope/1, P Scope/1, Sum/1
  P_shaft/1 -> P Scope/2, Sum/2
  Ix/1 -> Divide/3
  Constant/1 -> Ueo/2
  Ueo/1 -> Um/1
  Product1/1 -> Um/2
  Constant1/1 -> Product1/1
  Um/1 -> Ea/1
  Product2/1 -> Ea/2
  Constant2/1 -> Product2/1
  Ea/1 -> N(rpm)/1
  Constant3/1 -> N(rpm)/2
  Diameter/1 -> J/2
  V/1 -> J/1
  N(rpm)/1 -> Gain3/1, RPM 4/2
  J/1 -> Scope1/1, get CP/1
  theta_b/1 -> get CP/2
  Gain4/1 -> Q/2  "CQ"
  D^5/1 -> Math Function4/2
  Diameter1/1 -> Math Function4/1
  Math Function/1 -> Q/3  "n^2"
  Q/1 -> N(rpm)1/2
  Constant4/1 -> N(rpm)1/1
  N(rpm)1/1 -> Im/1
  Constant5/1 -> Im/2
  Im/1 -> Product1/2, Product2/2
  rho/1 -> Q/1, P_sp/3  "rho"
  Math Function3/1 -> P_sp/2  "n^3"
  "n^3 "/1 -> Math Function3/2
  Math Function4/1 -> Q/4, P_sp/4  "D^5"
  get CP/1 -> Gain4/1, Scope2/1, P_sp/1  "CP"
  Constant6/1 -> Manual Switch/2
  Manual Switch/1 -> Gain2/1
  Gain3/1 -> Memory/1
  Memory/1 -> J/3, Math Function3/1, Math Function/1

== system eVTOL_HIL/eVTOL Dynamic Model/Energy & Power/thrust_4/Propeller  ==
  rpm : Inport
  V : Inport  Port=2
  rho : Inport  Port=3
  theta_b : Inport  Port=4
  D^5 : Constant  Value=5
  Diameter : Constant  Value=Prop.D
  Divide : Product  Inputs=4
  Divide2 : Product  Inputs=4
  Divide3 : Product  Inputs=**/
  Gain : Gain  Gain=1/60
  Math Function : Math  Operator=magnitude^2  SignedPower=on
  Math Function1 : Math  Operator=magnitude^2  SignedPower=on
  Math Function2 : Math  Operator=magnitude^2  SignedPower=on
  Math Function3 : Math  Operator=pow  SignedPower=on
  Math Function4 : Math  Operator=pow  SignedPower=on
  Scope{,1..4} (5 alike) : Scope
  Subsystem : Subsystem
  get CP : Lookup_n-D  BreakpointsForDimension1=Prop.J  BreakpointsForDimension2=Prop.theta_b  IndexSearchMethod=Linear search  BeginIndexSearchUsingPreviousIndexResult=on  Table=Prop.CP  RndMeth=Simplest
      settings: InputPortMap=u0,u1
  get CT : Lookup_n-D  BreakpointsForDimension1=Prop.J  BreakpointsForDimension2=Prop.theta_b  IndexSearchMethod=Linear search  BeginIndexSearchUsingPreviousIndexResult=on  Table=Prop.CT  RndMeth=Simplest
      settings: InputPortMap=u0,u1
  "n^3 " : Constant  Value=3
  P_plr (w) : Outport  VectorParamsAs1DForOutWhenUnconnected=off
  T (N) : Outport  Port=2  VectorParamsAs1DForOutWhenUnconnected=off
  eta_p : Outport  Port=3  VectorParamsAs1DForOutWhenUnconnected=off
  wires:
  Divide2/1 -> P_plr (w)/1, Scope/1
  Divide3/1 -> eta_p/1  "eta_p"
  D^5/1 -> Math Function4/2
  Math Function4/1 -> Divide2/4
  "n^3 "/1 -> Math Function3/2
  Math Function3/1 -> Divide2/3
  get CP/1 -> Divide3/3, Divide2/1, Scope3/1
  rpm/1 -> Gain/1, Subsystem/2(rpm)
  Subsystem/1(J) -> Scope2/1, get CT/1, Divide3/1, get CP/1
  Divide/1 -> Scope1/1, T (N)/1
  Math Function2/1 -> Divide/4  "D^4"
  Math Function1/1 -> Math Function2/1
  Diameter/1 -> Math Function1/1, Math Function4/1
  Math Function/1 -> Divide/3  "n^2"
  Gain/1 -> Math Function3/1, Math Function/1
  rho/1 -> Divide/2, Divide2/2
  get CT/1 -> Divide3/2, Divide/1, Scope4/1
  V/1 -> Subsystem/1(V)
  theta_b/1 -> get CP/2, get CT/2

== system eVTOL_HIL/eVTOL Dynamic Model/Energy & Power/thrust_5/Motor ==
  P_shaft : Inport
  dt : Inport  Port=2
  V : Inport  Port=3
  rpm0 : Inport  Port=4
  rho : Inport  Port=5
  theta_b : Inport  Port=6
  Constant : Constant  Value=Motor.Ue
  Constant1 : Constant  Value=Motor.Re
  Constant2 : Constant  Value=Motor.Rm
  Constant3 : Constant  Value=Motor.KE
  Constant4 : Constant  Value=Motor.KT  VectorParams1D=off
  Constant5 : Constant  Value=Motor.Im0
  Constant6 : Constant  Value=0
  D^5 : Constant  Value=5
  Diameter : Constant  Value=Prop.D
  Diameter1 : Constant  Value=Prop.D
  Divide : Product  Inputs=*//
  Ea : Sum  Inputs=+-
  Gain1 : Gain  Gain=30/pi
  Gain2 : Gain  Gain=pi/30
  Gain3 : Gain  Gain=1/60
  Gain4 : Gain  Gain=1/(2*pi)
  Im : Sum
  Integrator : Integrator  InitialConditionSource=external  InitialCondition=600
  Ix : Constant  Value=Prop.Ix
  J : Product  Inputs=*//
  Manual Switch : ManualSwitch
  Math Function : Math  Operator=magnitude^2  SignedPower=on
  Math Function3 : Math  Operator=pow  SignedPower=on
  Math Function4 : Math  Operator=pow  SignedPower=on
  Memory : Memory  InitialCondition=0.1
  N(rpm) : Product  Inputs=*/
  N(rpm)1 : Product  Inputs=/*
  P Scope : Scope  NumInputPorts=2
  P_sp : Product  Inputs=4
  Product1 : Product
  Product2 : Product
  Q : Product  Inputs=4
  RPM 5 : Scope
  Saturation : Saturate  UpperLimit=104.72  LowerLimit=0.1
  Scope : Scope
  Sum : Sum  Inputs=|+-
  Ueo : Product
  Um : Sum  Inputs=+-
  get CP : Lookup_n-D  BreakpointsForDimension1=Prop.J  BreakpointsForDimension2=Prop.theta_b  IndexSearchMethod=Linear search  BeginIndexSearchUsingPreviousIndexResult=on  Table=Prop.CP  RndMeth=Simplest
      settings: InputPortMap=u0,u1
  "n^3 " : Constant  Value=3
  rpm : Outport  VectorParamsAs1DForOutWhenUnconnected=off
  wires:
  Saturation/1 -> Gain1/1, Divide/2
  Gain2/1 -> Integrator/2
  rpm0/1 -> Manual Switch/1
  Gain1/1 -> rpm/1, RPM 5/1  "rpm"
  Sum/1 -> Divide/1  "DP"
  Divide/1 -> Integrator/1  "omega_dot"
  dt/1 -> Ueo/1
  Integrator/1 -> Saturation/1  "omega"
  P_sp/1 -> Scope/1, P Scope/1, Sum/1
  P_shaft/1 -> P Scope/2, Sum/2
  Ix/1 -> Divide/3
  Constant/1 -> Ueo/2
  Ueo/1 -> Um/1
  Product1/1 -> Um/2
  Constant1/1 -> Product1/1
  Um/1 -> Ea/1
  Product2/1 -> Ea/2
  Constant2/1 -> Product2/1
  Ea/1 -> N(rpm)/1
  Constant3/1 -> N(rpm)/2
  Diameter/1 -> J/2
  V/1 -> J/1
  N(rpm)/1 -> Gain3/1
  J/1 -> get CP/1
  theta_b/1 -> get CP/2
  Gain4/1 -> Q/2  "CQ"
  D^5/1 -> Math Function4/2
  Diameter1/1 -> Math Function4/1
  Math Function/1 -> Q/3  "n^2"
  Q/1 -> N(rpm)1/2
  Constant4/1 -> N(rpm)1/1
  N(rpm)1/1 -> Im/1
  Constant5/1 -> Im/2
  Im/1 -> Product1/2, Product2/2
  rho/1 -> Q/1, P_sp/3  "rho"
  Math Function3/1 -> P_sp/2  "n^3"
  "n^3 "/1 -> Math Function3/2
  Math Function4/1 -> Q/4, P_sp/4  "D^5"
  get CP/1 -> Gain4/1, P_sp/1  "CP"
  Constant6/1 -> Manual Switch/2
  Manual Switch/1 -> Gain2/1
  Gain3/1 -> Memory/1  "rps"
  Memory/1 -> J/3, Math Function3/1, Math Function/1

== system eVTOL_HIL/eVTOL Dynamic Model/Energy & Power/thrust_5/Propeller  ==
  rpm : Inport
  V : Inport  Port=2
  rho : Inport  Port=3
  theta_b : Inport  Port=4
  D^5 : Constant  Value=5
  Diameter : Constant  Value=Prop.D
  Divide : Product  Inputs=4
  Divide2 : Product  Inputs=4
  Divide3 : Product  Inputs=**/
  Gain : Gain  Gain=1/60
  Math Function : Math  Operator=magnitude^2  SignedPower=on
  Math Function1 : Math  Operator=magnitude^2  SignedPower=on
  Math Function2 : Math  Operator=magnitude^2  SignedPower=on
  Math Function3 : Math  Operator=pow  SignedPower=on
  Math Function4 : Math  Operator=pow  SignedPower=on
  Scope{,1..4} (5 alike) : Scope
  Subsystem : Subsystem
  get CP : Lookup_n-D  BreakpointsForDimension1=Prop.J  BreakpointsForDimension2=Prop.theta_b  IndexSearchMethod=Linear search  BeginIndexSearchUsingPreviousIndexResult=on  Table=Prop.CP  RndMeth=Simplest
      settings: InputPortMap=u0,u1
  get CT : Lookup_n-D  BreakpointsForDimension1=Prop.J  BreakpointsForDimension2=Prop.theta_b  IndexSearchMethod=Linear search  BeginIndexSearchUsingPreviousIndexResult=on  Table=Prop.CT  RndMeth=Simplest
      settings: InputPortMap=u0,u1
  "n^3 " : Constant  Value=3
  P_plr (w) : Outport  VectorParamsAs1DForOutWhenUnconnected=off
  T (N) : Outport  Port=2  VectorParamsAs1DForOutWhenUnconnected=off
  eta_p : Outport  Port=3  VectorParamsAs1DForOutWhenUnconnected=off
  wires:
  Divide2/1 -> P_plr (w)/1, Scope/1
  Divide3/1 -> eta_p/1  "eta_p"
  D^5/1 -> Math Function4/2
  Math Function4/1 -> Divide2/4
  "n^3 "/1 -> Math Function3/2
  Math Function3/1 -> Divide2/3
  get CP/1 -> Divide3/3, Divide2/1, Scope3/1
  rpm/1 -> Gain/1, Subsystem/2(rpm)
  Subsystem/1(J) -> Scope2/1, get CT/1, Divide3/1, get CP/1
  Divide/1 -> Scope1/1, T (N)/1
  Math Function2/1 -> Divide/4  "D^4"
  Math Function1/1 -> Math Function2/1
  Diameter/1 -> Math Function1/1, Math Function4/1
  Math Function/1 -> Divide/3  "n^2"
  Gain/1 -> Math Function3/1, Math Function/1
  rho/1 -> Divide/2, Divide2/2
  get CT/1 -> Divide3/2, Divide/1, Scope4/1
  V/1 -> Subsystem/1(V)
  theta_b/1 -> get CP/2, get CT/2

== system eVTOL_HIL/eVTOL Dynamic Model/Energy & Power/thrust_6/Motor ==
  P_shaft : Inport
  dt : Inport  Port=2
  V : Inport  Port=3
  rpm0 : Inport  Port=4
  rho : Inport  Port=5
  theta_b : Inport  Port=6
  Constant : Constant  Value=Motor.Ue
  Constant1 : Constant  Value=Motor.Re
  Constant2 : Constant  Value=Motor.Rm
  Constant3 : Constant  Value=Motor.KE
  Constant4 : Constant  Value=Motor.KT  VectorParams1D=off
  Constant5 : Constant  Value=Motor.Im0
  Constant6 : Constant  Value=0
  D^5 : Constant  Value=5
  Diameter : Constant  Value=Prop.D
  Diameter1 : Constant  Value=Prop.D
  Divide : Product  Inputs=*//
  Ea : Sum  Inputs=+-
  Gain1 : Gain  Gain=30/pi
  Gain2 : Gain  Gain=pi/30
  Gain3 : Gain  Gain=1/60
  Gain4 : Gain  Gain=1/(2*pi)
  Im : Sum
  Integrator : Integrator  InitialConditionSource=external  InitialCondition=600
  Ix : Constant  Value=Prop.Ix
  J : Product  Inputs=*//
  Manual Switch : ManualSwitch
  Math Function : Math  Operator=magnitude^2  SignedPower=on
  Math Function3 : Math  Operator=pow  SignedPower=on
  Math Function4 : Math  Operator=pow  SignedPower=on
  Memory : Memory  InitialCondition=0.1
  N(rpm) : Product  Inputs=*/
  N(rpm)1 : Product  Inputs=/*
  P Scope : Scope  NumInputPorts=2
  P_sp : Product  Inputs=4
  Product1 : Product
  Product2 : Product
  Q : Product  Inputs=4
  RPM 6 : Scope
  Saturation : Saturate  UpperLimit=104.72  LowerLimit=0.1
  Scope : Scope
  Sum : Sum  Inputs=|+-
  Ueo : Product
  Um : Sum  Inputs=+-
  get CP : Lookup_n-D  BreakpointsForDimension1=Prop.J  BreakpointsForDimension2=Prop.theta_b  IndexSearchMethod=Linear search  BeginIndexSearchUsingPreviousIndexResult=on  Table=Prop.CP  RndMeth=Simplest
      settings: InputPortMap=u0,u1
  "n^3 " : Constant  Value=3
  rpm : Outport  VectorParamsAs1DForOutWhenUnconnected=off
  wires:
  Saturation/1 -> Gain1/1, Divide/2
  Gain2/1 -> Integrator/2
  rpm0/1 -> Manual Switch/1
  Gain1/1 -> rpm/1, RPM 6/1  "rpm"
  Sum/1 -> Divide/1  "DP"
  Divide/1 -> Integrator/1  "omega_dot"
  dt/1 -> Ueo/1
  Integrator/1 -> Saturation/1  "omega"
  P_sp/1 -> Scope/1, P Scope/1, Sum/1
  P_shaft/1 -> P Scope/2, Sum/2
  Ix/1 -> Divide/3
  Constant/1 -> Ueo/2
  Ueo/1 -> Um/1
  Product1/1 -> Um/2
  Constant1/1 -> Product1/1
  Um/1 -> Ea/1
  Product2/1 -> Ea/2
  Constant2/1 -> Product2/1
  Ea/1 -> N(rpm)/1
  Constant3/1 -> N(rpm)/2
  Diameter/1 -> J/2
  V/1 -> J/1
  N(rpm)/1 -> Gain3/1
  J/1 -> get CP/1
  theta_b/1 -> get CP/2
  Gain4/1 -> Q/2  "CQ"
  D^5/1 -> Math Function4/2
  Diameter1/1 -> Math Function4/1
  Math Function/1 -> Q/3  "n^2"
  Q/1 -> N(rpm)1/2
  Constant4/1 -> N(rpm)1/1
  N(rpm)1/1 -> Im/1
  Constant5/1 -> Im/2
  Im/1 -> Product1/2, Product2/2
  rho/1 -> Q/1, P_sp/3  "rho"
  Math Function3/1 -> P_sp/2  "n^3"
  "n^3 "/1 -> Math Function3/2
  Math Function4/1 -> Q/4, P_sp/4  "D^5"
  get CP/1 -> Gain4/1, P_sp/1  "CP"
  Constant6/1 -> Manual Switch/2
  Manual Switch/1 -> Gain2/1
  Gain3/1 -> Memory/1  "rps"
  Memory/1 -> J/3, Math Function3/1, Math Function/1
